simulink model "Passe_Bas"  (R2020a)
settings: Solver=VariableStepAuto  StartTime=0.0  StopTime=10  RelTol=1e-3
undefined symbols (not defined in the file): fdesignblkfcn, gcbh
libraries: dspspect3 x1, dspvision x1
settings Model: Creator=XPS 15  LastModifiedBy=XPS 15

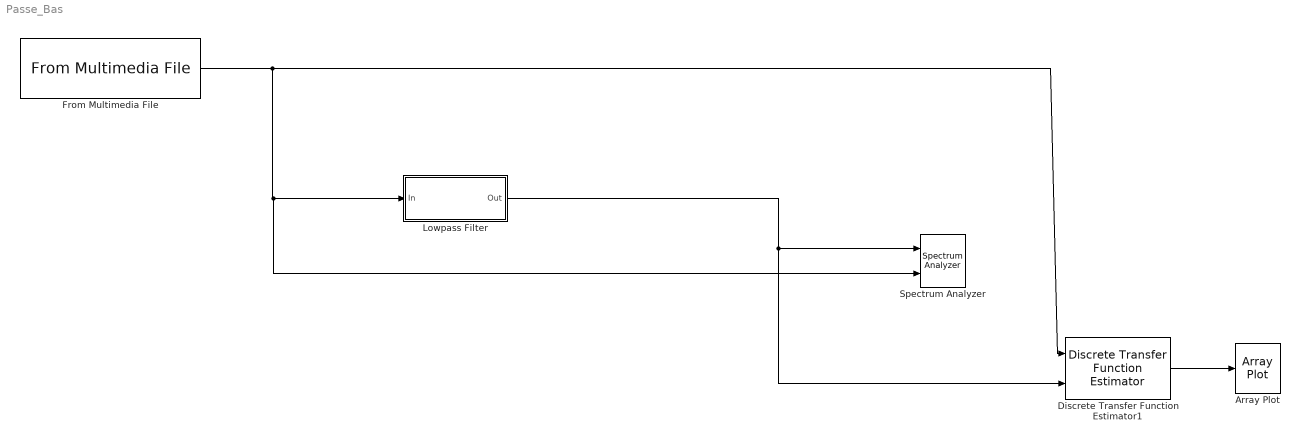
== system Passe_Bas ==
  Array Plot : ArrayPlot
  Discrete Transfer Function Estimator1 : dspspect3/Discrete Transfer Function Estimator  WindowMode=Specify on dialog  WindowLength=1024  Overlap=50  AveragingMethod=Running  ForgettingFactorPort=off  ForgettingFactor=0.9  SpectralAverages=100  FFTLengthSource=Auto  FFTLength=128  Window=Hann  SidelobeAttenuation=60  FrequencyRange=One-sided  OutputCoherence=off  SimulateUsing=Code generation
      settings: SourceProductBaseCode=DS
  From Multimedia File : dspvision/From Multimedia File  inputFilename=C:\Users\XPS 15\Desktop\L05 Sorbonne\images\Son\Projet\guitare.wav  readRange=[1 Inf]  loop=on  numPlays=inf  outputStreams=Audio only  videoDataType=single  audioDataType=double  inheritSampleTime=on  userDefinedSampleTime=1/30  noAudioOutput=off  isIntensityVideo=off  fourcc=RGB  colorVideoFormat=Separate color signals  outputEOF=off  dataOrg=Column-major  audioFrameSize=11025  computeAudioFrameSize=off  outSamplingMode=Sample based
  Lowpass Filter : Subsystem  DialogController=fdesignblkfcn  InitFcn=fdesignblkfcn(gcbh, {'InitFcn'});  mask(Lowpass Filter){}
      mask help: Design a lowpass filter
      settings: CopyFcn=fdesignblkfcn(gcbh, {'CopyFcn'});
      mask Help: helpview(mapfilelocation('dsp'), 'dsplowpassfilter');
      mask Display: disp('Lowpass')
  Spectrum Analyzer : SpectrumAnalyzer  NumInputPorts=2
  wires:
  Discrete Transfer Function Estimator1/1 -> Array Plot/1
  From Multimedia File/1 -> Discrete Transfer Function Estimator1/1, Spectrum Analyzer/2, Lowpass Filter/1(In)
  Lowpass Filter/1(Out) -> Spectrum Analyzer/1, Discrete Transfer Function Estimator1/2

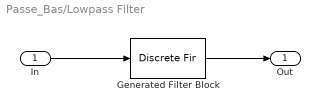
== system Passe_Bas/Lowpass Filter ==
  In : Inport
  Generated Filter Block : DiscreteFir  Tag=BlockMethodSubSystem  Coefficients=[-0.00249203399671605631 -0.00437214325754682609 -0.00196498725492353201 0.00109496478529590028 0.00526262897532535443 0.00432224555487157377 -0.000930143067547605667 -0.00755829918166998037 -0.00814332425845900112 -0.000591719043231979402 0.0102381876594105341 0.013721472538848891 0.0040548799688935799 -0.0129997110036866419 -0.0218735150379440052 -0.0107153117900186702 0.015546167756518136 0.0345894981822984157 0.0237177369869130024 -0.0176041953526959623 -0.0588900257169884811 -0.0553146647456019755 0.0189444450890528769 0.145239296105088345 0.264884125004560211 0.313923140972119541 0.264884125004560211 0.145239296105088345 0.0189444450890528769 -0.0553146647456019755 -0.0588900257169884811 -0.0176041953526959623 0.0237177369869130024 0.0345894981822984157 0.015546167756518136 -0.0107153117900186702 -0.0218735150379440052 -0.0129997110036866419 0.0040548799688935799 0.013721472538848891 0.0102381876594105341 -0.000591719043231979402 -0.00814332425845900112 -0.00755829918166998037 -0.000930143067547605667 0.00432224555487157377 0.00526262897532535443 0.00109496478529590028 -0.00196498725492353201 -0.00437214325754682609 -0.00249203399671605631]  InputProcessing=Columns as channels (frame based)
  Out : Outport
  wires:
  Generated Filter Block/1 -> Out/1
  In/1 -> Generated Filter Block/1
